simulink model "UTPR_MPC_LPV_22"  (R2023b)
settings: Solver=ode4  StartTime=0  StopTime=6  FixedStep=0.01  RelTol=1e-2  AbsTol=1e-3  EnableMultiTasking=on
values from neighbouring files (symbols this model uses):
  H = 0.05    [utpr_model_complex_para.m]    (also in utpr_mpc.m = (H + H')/2)
  L1 = 0.325    [utpr_model_complex_para.m]
  L2 = 0.2    [utpr_model_complex_para.m]
  L3 = 0.2    [utpr_model_complex_para.m]
  link1_CM = [245.436 * 1e-3 0 0]    [utpr_model_complex_para.m]
  link1_m = 1.915 * (rand_para(1,1) + 1)    [utpr_model_complex_para.m]
  link1_MI = [0 0 25720.752*1e-6* (rand_para(2,1) + 1)]    [utpr_model_complex_para.m]
  link1_PI = [0 0 0]    [utpr_model_complex_para.m]
  link2_CM = [165.468 * 1e-3 0 0]    [utpr_model_complex_para.m]
  link2_m = 1.469 * (rand_para(3,1) + 1)    [utpr_model_complex_para.m]
  link2_MI = [0 0 7667.511*1e-6* (rand_para(4,1) + 1)]    [utpr_model_complex_para.m]
  link2_PI = [0 0 0]    [utpr_model_complex_para.m]
  link3_CM = [127.337*1e-3 0 0]    [utpr_model_complex_para.m]
  link3_m = 1.141 * (rand_para(5,1) + 1)    [utpr_model_complex_para.m]
  link3_MI = [0 0 4949.014*1e-6* (rand_para(6,1) + 1)]    [utpr_model_complex_para.m]
  link3_PI = [0 0 0 ]    [utpr_model_complex_para.m]
  N = 50    [utpr_lqr.m]    (also in utpr_mpc.m = 100)
  W = 0.05    [utpr_model_complex_para.m]
undefined symbols (not defined in the file or in its folder): X, Y, Z
libraries: nesl_utility x24, sm_lib x17
settings Model: Creator=李东昊  LastModifiedBy=12720
settings SolverCC: AutoScaleAbsTol=off  AlgebraicLoopSolver=TrustRegion  MaxZcPerStep=1
settings DataIOCC: LimitDataPoints=on  MaxDataPoints=10000
settings OptimizationCC: ReuseModelBlockBuffer=off  LifeSpan=inf
settings DebuggingCC: UnconnectedInputMsg=warning  UnconnectedOutputMsg=warning  UnconnectedLineMsg=warning  AllowSymbolicDim=off  SFUnexpectedBacktrackingDiag=warning  SFNoUnconditionalDefaultTransitionDiag=warning  SFExecutionAtInitializationDiag=none  ArithmeticOperatorsInVariantConditions=warning
settings ModelReferenceCC: EnableRefExpFcnMdlSchedulingChecks=on
settings SFSimCC: SimUseLocalCustomCode=off  CustomCodeUndefinedFunction=UseInterfaceOnly
settings RTWCC: RTWUseLocalCustomCode=off  DLArmComputeVersion=19.05
settings CodeAppCC: StateflowObjectComments=on
settings GRTTargetCC: TargetLangStandard=C89/C90 (ANSI)
settings ConfigComp: CovMetricSettings=dw  CovSaveCumulativeToWorkspaceVar=on  CovSaveSingleToWorkspaceVar=on  CovExternalEMLEnable=off  CovSFcnEnable=off
settings SimscapeCC: SimscapeLogType=all  SimscapeLogSimulationStatistics=on  SimscapeLogDataHistory=10000
settings ExplorerConfigSet: InternalSimMechanicsExplorerSettings="<ExplorerConfiguration><canonicalview>aerospace</canonicalview><AnimationSetting><BasePlaybackSpeed>1.0</BasePlaybackSpeed><PlaybackSpeedFactor>1.0</PlaybackSpeedFactor></AnimationSetting><TilePanel><TileInfo><Tiles Columns=\"1\" Count=\"1\" Rows=\"1\"><Column Weight=\"1\"/><Row Weight=\"1\"/><Tile Height=\"1\" Width=\"1\" X=\"0\" Y=\"0\"/></Tiles></TileInfo><SceneInfo><SceneViewer><BGColor><R>0.60000002384185791</R><G>0.60000002384185791</G><B>0.60000002384185791</B></BGColor><Camera><DoPerspective>off</DoPerspective><Position><X>-0.471212034882517727</X><Y>0.213512906624389098</Y><Z>1.00000005247557366</Z></Position><Center><X>-0.471212034882517727</X><Y>0.213512906624389098</Y><Z>5.24755735531456935e-08</Z></Center><Up><X>0</X><Y>1</Y><Z>0</Z></Up><ViewLimDist>1</ViewLimDist><YLim>1.41406501065933288</YLim><XLim>1.62924881662923138</XLim></Camera></SceneViewer></SceneInfo></TilePanel><MechEditorPanel><Cameras/><GfxPanelCameraMap/><VideoCreator><PlaybackSpeedRatio>1.0</PlaybackSpeedRatio><FrameRate>30</FrameRate><VideoFormat>MPEG-4</VideoFormat><FrameSize>[800 600]</FrameSize></VideoCreator></MechEditorPanel></ExplorerConfiguration>"

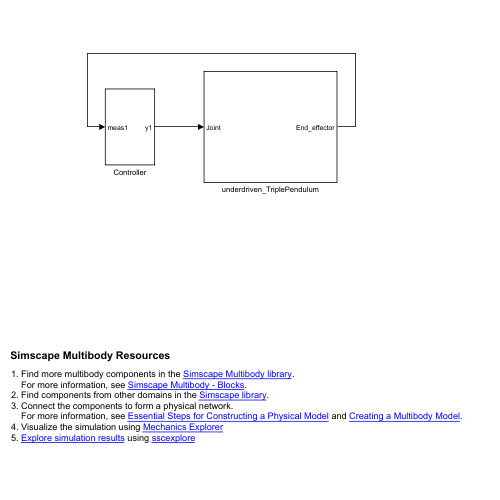
[thumbnail: Simulink's stored preview of the top-level diagram]
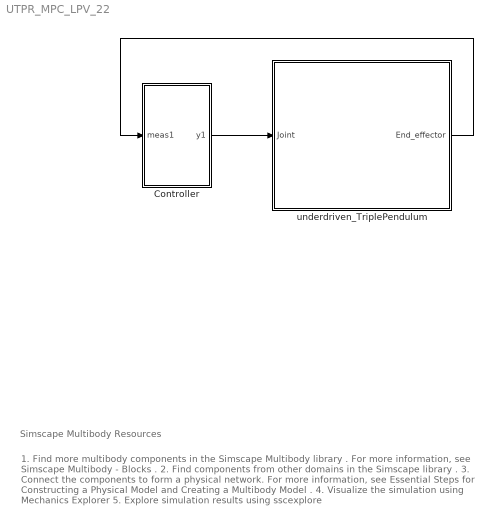
== system UTPR_MPC_LPV_22 ==
  note: 1. Find more multibody components in the Simscape Multibody library .
      | For more information, see Simscape Multibody - Blocks .
      | 2. Find components from other domains in the Simscape library .
      | 3. Connect the components to form a physical network.
      | For more information, see Essential Steps for Constructing a Physical Model and Creating a Multibody Model .
      | 4. Visualize the simulation using Mechanics Explorer
      | 5. Explore simulation results using sscexplore
  note: Simscape Multibody Resources
  Controller : Subsystem  Priority=1
  underdriven_TriplePendulum : Subsystem  Priority=2
  wires:
  underdriven_TriplePendulum/1(End_effector) -> Controller/1(meas1)
  Controller/1(y1) -> underdriven_TriplePendulum/1(Joint)

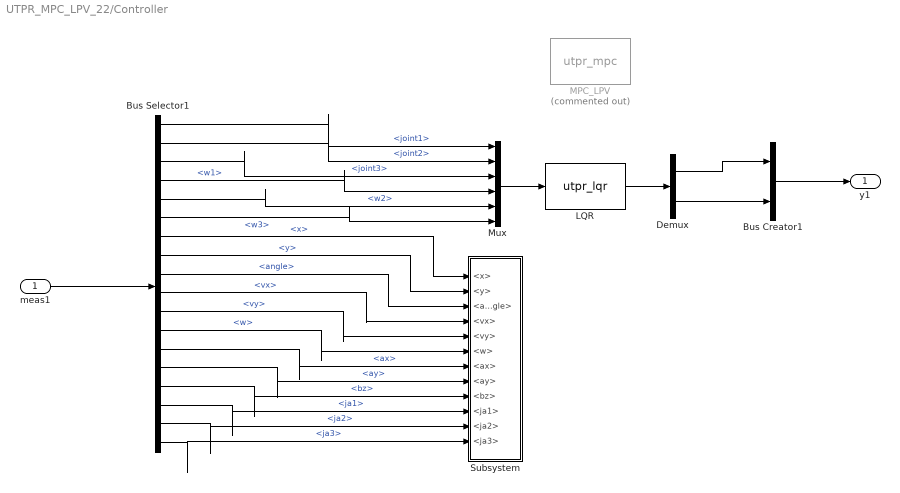
== system UTPR_MPC_LPV_22/Controller ==
  meas1 : Inport
  Bus Creator1 : BusCreator  Inputs=2
  Bus Selector1 : BusSelector  OutputSignals=joint1,joint2,joint3,w1,w2,w3,signal1.x,signal1.y,signal1.angle,signal1.vx,signal1.vy,signal1.w,signal1.ax,signal1.ay,signal1.bz,ja1,ja2,ja3
  Demux : Demux  Outputs=2
  LQR : MATLABFcn  MATLABFcn=utpr_lqr  OutputDimensions=2
  MPC_LPV : MATLABFcn  Commented=on  MATLABFcn=utpr_mpc  OutputDimensions=2
  Mux : Mux  Inputs=6
  Subsystem : Subsystem
  y1 : Outport
  wires:
  Bus Creator1/1 -> y1/1
  meas1/1 -> Bus Selector1/1
  Bus Selector1/1 -> Mux/1  "<joint1>"
  Bus Selector1/2 -> Mux/2  "<joint2>"
  Bus Selector1/3 -> Mux/3  "<joint3>"
  Bus Selector1/4 -> Mux/4  "<w1>"
  Bus Selector1/6 -> Mux/6  "<w3>"
  Demux/1 -> Bus Creator1/1
  Demux/2 -> Bus Creator1/2
  Bus Selector1/7 -> Subsystem/1(<x>)  "<x>"
  Bus Selector1/8 -> Subsystem/2(<y>)  "<y>"
  Bus Selector1/9 -> Subsystem/3(<angle>)  "<angle>"
  Bus Selector1/10 -> Subsystem/4(<vx>)  "<vx>"
  Bus Selector1/11 -> Subsystem/5(<vy>)  "<vy>"
  Bus Selector1/12 -> Subsystem/6(<w>)  "<w>"
  Bus Selector1/13 -> Subsystem/7(<ax>)  "<ax>"
  Bus Selector1/14 -> Subsystem/8(<ay>)  "<ay>"
  Bus Selector1/15 -> Subsystem/9(<bz>)  "<bz>"
  Bus Selector1/16 -> Subsystem/10(<ja1>)  "<ja1>"
  Bus Selector1/17 -> Subsystem/11(<ja2>)  "<ja2>"
  Bus Selector1/18 -> Subsystem/12(<ja3>)  "<ja3>"
  Bus Selector1/5 -> Mux/5  "<w2>"
  Mux/1 -> LQR/1
  LQR/1 -> Demux/1

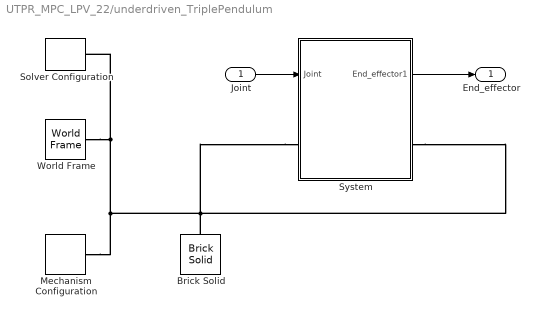
== system UTPR_MPC_LPV_22/underdriven_TriplePendulum ==
  Joint : Inport
  Brick Solid : sm_lib/Body Elements/Brick Solid  BrickDimensions=[0.1 0.1 0.1]  BrickDimensionsUnits=m  ExportEntireGeometry=off  InertiaType=CalculateFromGeometry  BasedOnType=Density  Density=1000  DensityUnits=kg/m^3  Mass=1  MassUnits=kg  CenterOfMass=[0 0 0]  CenterOfMassUnits=m  MomentsOfInertia=[1 1 1]  MomentsOfInertiaUnits=kg*m^2  ProductsOfInertia=[0 0 0]  ProductsOfInertiaUnits=kg*m^2  GraphicType=FromGeometry  MarkerShape=Sphere  MarkerSize=10  GraphicVisPropType=SimpleVisualProperties  GraphicDiffuseColor=[0.5 0.5 0.5]  GraphicOpacity=1.0  GraphicSpecularColor=[0.5 0.5 0.5 1.0]  GraphicAmbientColor=[0.15 0.15 0.15 1.0]  GraphicEmissiveColor=[0.0 0.0 0.0 1.0]  GraphicShininess=75  DoExposeReferenceFrame=on  SerializedFrames=<Frames/>
  Mechanism Configuration : sm_lib/Utilities/Mechanism Configuration  UniformGravity=Constant  GravityVector=[0 -9.81 0]  GravityVectorUnits=m/s^2  LinearizationDelta=0.001  JointModeTransitionNonlinearIterations=2
  Solver Configuration : nesl_utility/Solver Configuration  PhysicalDomain=network_engine_domain  SubClassName=solver  LeftPortType=input  RightPortType=generic  Tones=[]  Harmonics=[]  SimulateNoise=off  Profile=off  UseLocalSampling=off  EnableSwitchedLinearOptims=on  FrequencyDomain=off  UseCCode=off  RelTol=0.001  AbsTol=1e-06  MinStep=1e-09  ToWorkspace=off  RevertToSquareIcSolve=off  NumHomotopyIterations=100  PhasorMode=off  PhasorModeNumHarmonics=1  ConsistencySolver=NEWTON_FTOL  IndexReductionMethod=DerivativeReplacement  DoDC=off  ResidualTolerance=1e-09  ConsistencyTolSource=GLOBAL  ConsistencyAbsTol=0.001  ConsistencyRelTol=0.001  ConsistencyTolFactor=0.001  UseLocalSolver=off  LocalSolverChoice=NE_BACKWARD_EULER_ADVANCER  ResolveIndetEquations=on  FunctionEvalNumThread=1  LocalSolverSampleTime=0.001  DoFixedCost=off  MaxNonlinIter=3  MaxModeIter=2  ComputeImpulses=off  ImpulseIterations=2  LinearAlgebra=Sparse  LinearAlgebraNumThread=0  EquationFormulation=NE_TIME_EF  DelaysMemoryBudget=1024  AutomaticFiltering=on  FilteringTimeConstant=0.001  PartitionStorageMethod=AS_NEEDED  PartitionMemoryBudget=1024  PartitionMethod=FAST  MultibodyUseLocalSolver=off  MultibodyLocalSolverChoice=ODE1  MultibodyLocalSolverSampleTime=0.001
  System : Subsystem
  World Frame : sm_lib/Frames and Transforms/World Frame
  End_effector : Outport
  wires:
  Joint/1 -> System/1(Joint)
  System/1(End_effector1) -> End_effector/1
  connections:
  System/LConn1 -- World Frame/RConn1 -- Solver Configuration/RConn1 -- Mechanism Configuration/RConn1 -- Brick Solid/RConn1 -- System/RConn1

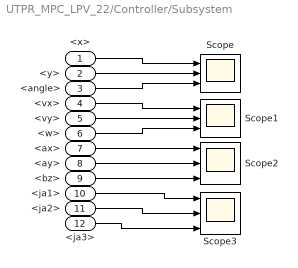
== system UTPR_MPC_LPV_22/Controller/Subsystem ==
  <x> : Inport
  <y> : Inport  Port=2
  <angle> : Inport  Port=3
  <vx> : Inport  Port=4
  <vy> : Inport  Port=5
  <w> : Inport  Port=6
  <ax> : Inport  Port=7
  <ay> : Inport  Port=8
  <bz> : Inport  Port=9
  <ja1> : Inport  Port=10
  <ja2> : Inport  Port=11
  <ja3> : Inport  Port=12
  Scope{,1..3} (4 alike) : Scope  NumInputPorts=3
  wires:
  <y>/1 -> Scope/2
  <ja1>/1 -> Scope3/1
  <bz>/1 -> Scope2/3
  <ax>/1 -> Scope2/1
  <vy>/1 -> Scope1/2
  <x>/1 -> Scope/1
  <angle>/1 -> Scope/3
  <ja2>/1 -> Scope3/2
  <ay>/1 -> Scope2/2
  <w>/1 -> Scope1/3
  <vx>/1 -> Scope1/1
  <ja3>/1 -> Scope3/3

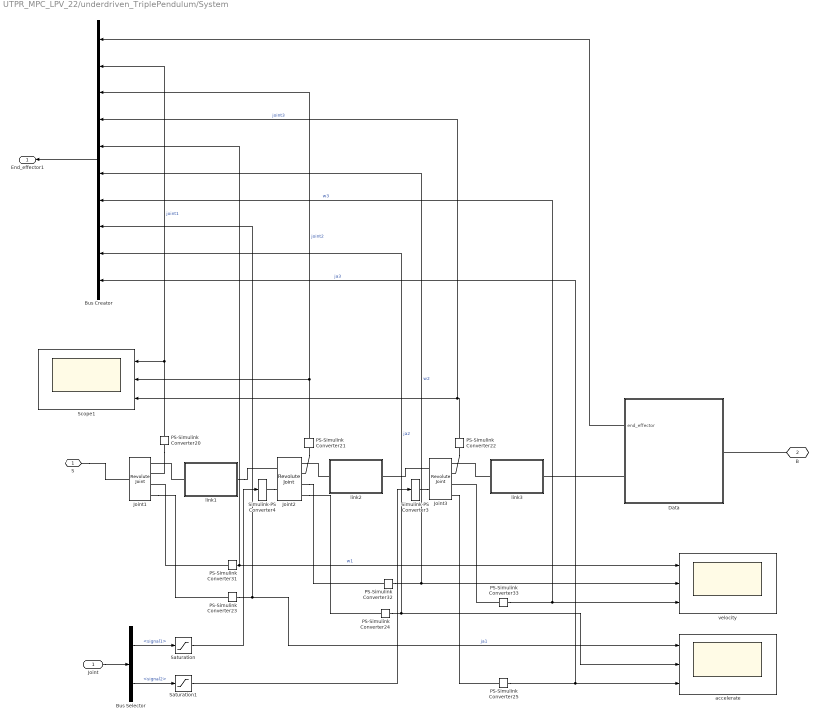
== system UTPR_MPC_LPV_22/underdriven_TriplePendulum/System ==
  Joint : Inport
  Bus Creator : BusCreator  Inputs=10
  Bus Selector : BusSelector  OutputSignals=signal1,signal2
  Data : Subsystem
  Joint1 : sm_lib/Joints/Revolute Joint  JointMode=Normal  CompositeWrenchDir=BaseOnFollower  CompositeWrenchFrame=BaseFrame  SenseConstraintForce=off  SenseConstraintTorque=off  SenseTotalForce=off  SenseTotalTorque=off  PositionTargetSpecify=on  PositionTargetPriority=High  PositionTargetValue=0.9  PositionTargetValueUnits=deg  VelocityTargetSpecify=off  VelocityTargetPriority=Low  VelocityTargetValue=0  VelocityTargetValueUnits=rad/s  EquilibriumPosition=0  EquilibriumPositionUnits=deg  SpringStiffness=0  SpringStiffnessUnits=N*m/deg  DampingCoefficient=0  DampingCoefficientUnits=N*m/(deg/s)  LowerLimitSpecify=off  LowerLimitBound=-90  LowerLimitBoundUnits=deg  LowerLimitStiffness=1e4  LowerLimitStiffnessUnits=N*m/deg  LowerLimitDamping=10  LowerLimitDampingUnits=N*m/(deg/s)  LowerLimitTransitionRegionWidth=0.1  LowerLimitTransitionRegionWidthUnits=deg  UpperLimitSpecify=off  UpperLimitBound=90  UpperLimitBoundUnits=deg  UpperLimitStiffness=1e4  UpperLimitStiffnessUnits=N*m/deg  UpperLimitDamping=10  UpperLimitDampingUnits=N*m/(deg/s)  UpperLimitTransitionRegionWidth=0.1  UpperLimitTransitionRegionWidthUnits=deg  TorqueActuationMode=NoTorque  MotionActuationMode=ComputedMotion  SensePosition=on  SenseVelocity=on  SenseAcceleration=on  SenseTorqueForce=off  SenseLowerLimitTorqueForce=off  SenseUpperLimitTorqueForce=off
  Joint2 : sm_lib/Joints/Revolute Joint  JointMode=Normal  CompositeWrenchDir=BaseOnFollower  CompositeWrenchFrame=BaseFrame  SenseConstraintForce=off  SenseConstraintTorque=off  SenseTotalForce=off  SenseTotalTorque=off  PositionTargetSpecify=on  PositionTargetPriority=High  PositionTargetValue=0.9  PositionTargetValueUnits=deg  VelocityTargetSpecify=off  VelocityTargetPriority=High  VelocityTargetValue=0  VelocityTargetValueUnits=rad/s  EquilibriumPosition=0  EquilibriumPositionUnits=deg  SpringStiffness=0  SpringStiffnessUnits=N*m/deg  DampingCoefficient=0  DampingCoefficientUnits=N*m/(deg/s)  LowerLimitSpecify=off  LowerLimitBound=-90  LowerLimitBoundUnits=rad  LowerLimitStiffness=0  LowerLimitStiffnessUnits=N*m/deg  LowerLimitDamping=0  LowerLimitDampingUnits=N*m/(deg/s)  LowerLimitTransitionRegionWidth=0.0  LowerLimitTransitionRegionWidthUnits=deg  UpperLimitSpecify=off  UpperLimitBound=90  UpperLimitBoundUnits=deg  UpperLimitStiffness=1e4  UpperLimitStiffnessUnits=N*m/deg  UpperLimitDamping=10  UpperLimitDampingUnits=N*m/(deg/s)  UpperLimitTransitionRegionWidth=0.1  UpperLimitTransitionRegionWidthUnits=deg  TorqueActuationMode=InputTorque  MotionActuationMode=ComputedMotion  SensePosition=on  SenseVelocity=on  SenseAcceleration=on  SenseTorqueForce=off  SenseLowerLimitTorqueForce=off  SenseUpperLimitTorqueForce=off
  Joint3 : sm_lib/Joints/Revolute Joint  JointMode=Normal  CompositeWrenchDir=BaseOnFollower  CompositeWrenchFrame=BaseFrame  SenseConstraintForce=off  SenseConstraintTorque=off  SenseTotalForce=off  SenseTotalTorque=off  PositionTargetSpecify=on  PositionTargetPriority=High  PositionTargetValue=0.9  PositionTargetValueUnits=deg  VelocityTargetSpecify=off  VelocityTargetPriority=High  VelocityTargetValue=0  VelocityTargetValueUnits=rad/s  EquilibriumPosition=0  EquilibriumPositionUnits=deg  SpringStiffness=0  SpringStiffnessUnits=N*m/deg  DampingCoefficient=0  DampingCoefficientUnits=N*m/(deg/s)  LowerLimitSpecify=off  LowerLimitBound=-90  LowerLimitBoundUnits=deg  LowerLimitStiffness=1e4  LowerLimitStiffnessUnits=N*m/deg  LowerLimitDamping=10  LowerLimitDampingUnits=N*m/(deg/s)  LowerLimitTransitionRegionWidth=0.1  LowerLimitTransitionRegionWidthUnits=deg  UpperLimitSpecify=off  UpperLimitBound=90  UpperLimitBoundUnits=deg  UpperLimitStiffness=1e4  UpperLimitStiffnessUnits=N*m/deg  UpperLimitDamping=10  UpperLimitDampingUnits=N*m/(deg/s)  UpperLimitTransitionRegionWidth=0.1  UpperLimitTransitionRegionWidthUnits=deg  TorqueActuationMode=InputTorque  MotionActuationMode=ComputedMotion  SensePosition=on  SenseVelocity=on  SenseAcceleration=on  SenseTorqueForce=off  SenseLowerLimitTorqueForce=off  SenseUpperLimitTorqueForce=off
  PS-Simulink Converter{20..25,31..33} (9 alike) : nesl_utility/PS-Simulink Converter  PhysicalDomain=network_engine_domain  SubClassName=ps_output  LeftPortType=input  RightPortType=output  PseudoPeriodic=off  Frequencies=[]  VectorFormat=inherit  Unit=inherit  AffineConversion=off
  Saturation : Saturate  UpperLimit=3  LowerLimit=-3
  Saturation1 : Saturate  UpperLimit=3  LowerLimit=-3
  Scope1 : Scope  NumInputPorts=3
  Simulink-PS Converter3 : nesl_utility/Simulink-PS Converter  PhysicalDomain=network_engine_domain  SubClassName=ps_input  LeftPortType=input  RightPortType=output  PseudoPeriodic=off  Frequencies=[]  NoiseDistribution=none  NoiseParameters=[]  Unit=1  AffineConversion=off  FilteringAndDerivatives=provide  SimscapeFilterOrder=2  InputFilterTimeConstant=0.001  UdotUserProvided=0
  Simulink-PS Converter4 : nesl_utility/Simulink-PS Converter  PhysicalDomain=network_engine_domain  SubClassName=ps_input  LeftPortType=input  RightPortType=output  PseudoPeriodic=off  Frequencies=[]  NoiseDistribution=none  NoiseParameters=[]  Unit=1  AffineConversion=off  FilteringAndDerivatives=provide  SimscapeFilterOrder=2  InputFilterTimeConstant=0.001  UdotUserProvided=0
  accelerate : Scope  NumInputPorts=3
  link1 : Subsystem  mask{L=L1, H=H, W=W, m=link1_m, link1_CM=link1_CM, link1_MI=link1_MI, link1_PI=link1_PI, rgb=[0.2 0.3 0.4]}
      mask prompts: link1_CM "Center of Mass"; link1_MI "Moments of Inertia"; link1_PI "Products of Inertia"; rgb "Color"
      mask DialogControl ParameterGroupVar Prompt: 参数
  link2 : Subsystem  mask{L=L2, W=W, H=W, llink2_m=link2_m, link2_CM=link2_CM, link2_MI=link2_MI, link2_PI=link2_PI, rgb=[1 1 0]}
      mask prompts: llink2_m "m(kg)"; link2_CM "Center of Mass"; link2_MI "Moments of Inertia"; link2_PI "Products of Inertia"
      mask DialogControl ParameterGroupVar Prompt: 参数
  link3 : Subsystem  mask{L=L3, W=W, H=H, link3_m=link3_m, link3_CM=link3_CM, link3_MI=link3_MI, link3_PI=link3_PI, rgb=[1 0.40 0.00]}
      mask prompts: link3_m "m"; link3_CM "Center of Mass"; link3_MI "Moments of Inertia"; link3_PI "Product of Inertia"
      mask DialogControl ParameterGroupVar Prompt: 参数
  velocity : Scope  NumInputPorts=3
  S : PMIOPort  Side=Left
  B : PMIOPort  Port=2  Side=Right
  End_effector1 : Outport
  wires:
  PS-Simulink Converter24/1 -> accelerate/2, Bus Creator/9  "ja2"
  PS-Simulink Converter32/1 -> Bus Creator/6, velocity/2  "w2"
  PS-Simulink Converter25/1 -> Bus Creator/10, accelerate/3  "ja3"
  PS-Simulink Converter22/1 -> Bus Creator/4, Scope1/3  "joint3"
  PS-Simulink Converter20/1 -> Bus Creator/2, Scope1/1  "joint1"
  Bus Selector/2 -> Saturation1/1  "<signal2>"
  PS-Simulink Converter21/1 -> Bus Creator/3, Scope1/2  "joint2"
  Bus Selector/1 -> Saturation/1  "<signal1>"
  PS-Simulink Converter33/1 -> Bus Creator/7, velocity/3  "w3"
  PS-Simulink Converter31/1 -> Bus Creator/5, velocity/1  "w1"
  Joint/1 -> Bus Selector/1
  Data/1(end_effector) -> Bus Creator/1
  Bus Creator/1 -> End_effector1/1
  PS-Simulink Converter23/1 -> accelerate/1, Bus Creator/8  "ja1"
  Saturation/1 -> Simulink-PS Converter4/1
  Saturation1/1 -> Simulink-PS Converter3/1
  connections:
  PS-Simulink Converter21/LConn1 -- Joint2/RConn2
  Joint2/RConn4 -- PS-Simulink Converter24/LConn1
  Joint3/RConn4 -- PS-Simulink Converter25/LConn1
  PS-Simulink Converter20/LConn1 -- Joint1/RConn2
  link1/LConn1 -- Joint1/RConn1
  PS-Simulink Converter22/LConn1 -- Joint3/RConn2
  link1/RConn1 -- Joint2/LConn1
  Simulink-PS Converter3/RConn1 -- Joint3/LConn2
  Joint1/RConn4 -- PS-Simulink Converter23/LConn1
  PS-Simulink Converter33/LConn1 -- Joint3/RConn3
  PS-Simulink Converter31/LConn1 -- Joint1/RConn3
  link3/LConn1 -- Joint3/RConn1
  S/RConn1 -- Joint1/LConn1
  link2/LConn1 -- Joint2/RConn1
  Joint3/LConn1 -- link2/RConn1
  Simulink-PS Converter4/RConn1 -- Joint2/LConn2
  Joint2/RConn3 -- PS-Simulink Converter32/LConn1
  B/RConn1 -- Data/LConn1
  Data/RConn1 -- link3/RConn1

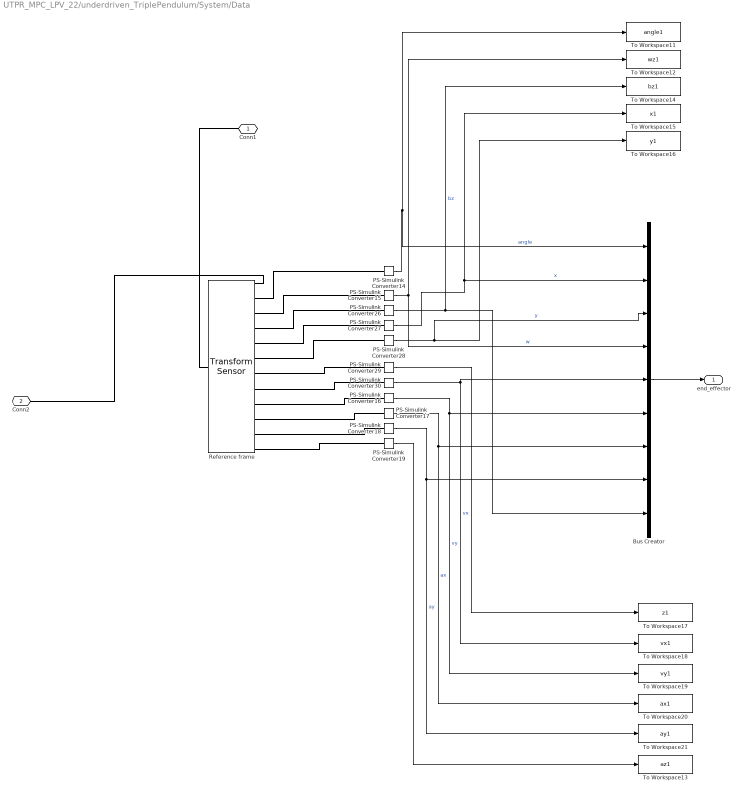
== system UTPR_MPC_LPV_22/underdriven_TriplePendulum/System/Data ==
  Bus Creator : BusCreator  Inputs=9
  PS-Simulink Converter{14..19,26..30} (11 alike) : nesl_utility/PS-Simulink Converter  PhysicalDomain=network_engine_domain  SubClassName=ps_output  LeftPortType=input  RightPortType=output  PseudoPeriodic=off  Frequencies=[]  VectorFormat=inherit  Unit=inherit  AffineConversion=off
  Reference frame : sm_lib/Frames and Transforms/Transform Sensor  MeasurementFrame=Base  RotationSequence=XYX  SenseAngle=on  SenseAxis=off  SenseQ=off  SenseR=off  SenseRotationSequence=off  SenseOmegaX=off  SenseOmegaY=off  SenseOmegaZ=on  SenseOmega=off  SenseQDot=off  SenseRDot=off  SenseRotationSequenceDot=off  SenseAlphaX=off  SenseAlphaY=off  SenseAlphaZ=on  SenseAlpha=off  SenseQDDot=off  SenseRDDot=off  SenseX=on  SenseY=on  SenseZ=on  SenseXYZ=off  SenseRad=off  SenseAzim=off  SenseDist=off  SenseInc=off  SenseXDot=on  SenseYDot=on  SenseZDot=off  SenseXYZDot=off  SenseRadDot=off  SenseAzimDot=off  SenseDistDot=off  SenseIncDot=off  SenseXDDot=on  SenseYDDot=on  SenseZDDot=on  SenseXYZDDot=off  SenseRadDDot=off  SenseAzimDDot=off  SenseDistDDot=off  SenseIncDDot=off
  To Workspace11 : ToWorkspace  VariableName=angle1  SaveFormat=Structure With Time  SampleTime=-1
  To Workspace12 : ToWorkspace  VariableName=wz1  SaveFormat=Structure With Time  SampleTime=-1
  To Workspace13 : ToWorkspace  VariableName=az1  SaveFormat=Structure With Time  SampleTime=-1
  To Workspace14 : ToWorkspace  VariableName=bz1  SaveFormat=Structure With Time  SampleTime=-1
  To Workspace15 : ToWorkspace  VariableName=x1  SaveFormat=Structure With Time  SampleTime=-1
  To Workspace16 : ToWorkspace  VariableName=y1  SaveFormat=Structure With Time  SampleTime=-1
  To Workspace17 : ToWorkspace  VariableName=z1  SaveFormat=Structure With Time  SampleTime=-1
  To Workspace18 : ToWorkspace  VariableName=vx1  SaveFormat=Structure With Time  SampleTime=-1
  To Workspace19 : ToWorkspace  VariableName=vy1  SaveFormat=Structure With Time  SampleTime=-1
  To Workspace20 : ToWorkspace  VariableName=ax1  SaveFormat=Structure With Time  SampleTime=-1
  To Workspace21 : ToWorkspace  VariableName=ay1  SaveFormat=Structure With Time  SampleTime=-1
  Conn1 : PMIOPort  Side=Left
  Conn2 : PMIOPort  Port=2  Side=Right
  end_effector : Outport
  wires:
  PS-Simulink Converter26/1 -> Bus Creator/9, To Workspace14/1  "bz"
  PS-Simulink Converter17/1 -> Bus Creator/7, To Workspace20/1  "ax"
  PS-Simulink Converter18/1 -> Bus Creator/8, To Workspace21/1  "ay"
  PS-Simulink Converter15/1 -> To Workspace12/1, Bus Creator/4  "w"
  PS-Simulink Converter27/1 -> Bus Creator/2, To Workspace15/1  "x"
  PS-Simulink Converter29/1 -> To Workspace17/1
  PS-Simulink Converter19/1 -> To Workspace13/1
  PS-Simulink Converter14/1 -> Bus Creator/1, To Workspace11/1  "angle"
  PS-Simulink Converter16/1 -> To Workspace19/1, Bus Creator/6  "vy"
  PS-Simulink Converter28/1 -> To Workspace16/1, Bus Creator/3  "y"
  PS-Simulink Converter30/1 -> To Workspace18/1, Bus Creator/5  "vx"
  Bus Creator/1 -> end_effector/1
  connections:
  Reference frame/RConn3 -- PS-Simulink Converter15/LConn1
  Reference frame/RConn7 -- PS-Simulink Converter29/LConn1
  Reference frame/RConn6 -- PS-Simulink Converter28/LConn1
  Reference frame/RConn8 -- PS-Simulink Converter30/LConn1
  Reference frame/RConn9 -- PS-Simulink Converter16/LConn1
  Reference frame/RConn11 -- PS-Simulink Converter18/LConn1
  Reference frame/RConn4 -- PS-Simulink Converter26/LConn1
  PS-Simulink Converter14/LConn1 -- Reference frame/RConn2
  Reference frame/RConn10 -- PS-Simulink Converter17/LConn1
  Reference frame/RConn5 -- PS-Simulink Converter27/LConn1
  Reference frame/RConn1 -- Conn2/RConn1
  Conn1/RConn1 -- Reference frame/LConn1
  Reference frame/RConn12 -- PS-Simulink Converter19/LConn1

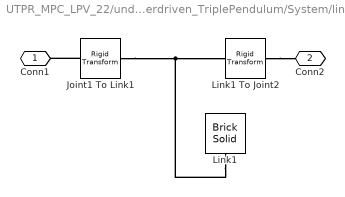
== system UTPR_MPC_LPV_22/underdriven_TriplePendulum/System/link1 ==
  Joint1 To Link1 : sm_lib/Frames and Transforms/Rigid Transform  RotationMethod=StandardAxis  FollAlignAxisA=+X  BaseAlignAxisA=+Y  FollAlignAxisB=+Y  BaseAlignAxisB=+Z  RotationStandardAxis=+Z  RotationAngle=90  RotationAngleUnits=deg  RotationArbitraryAxis=[0 0 1]  RotationSequenceAxes=FollowerAxes  RotationSequence=XYX  RotationSequenceAngles=[0 0 0]  RotationSequenceAnglesUnits=deg  RotationMatrix=[1 0 0; 0 1 0; 0 0 1]  Quaternion=[1 0 0 0]  TranslationMethod=StandardAxis  TranslationCartesianOffset=[0 0 0]  TranslationCartesianOffsetUnits=m  TranslationStandardAxis=+Y  TranslationStandardOffset=0  TranslationStandardOffsetUnits=m  TranslationROffset=0  TranslationROffsetUnits=m  TranslationThetaOffset=0  TranslationThetaOffsetUnits=deg  TranslationZOffset=0  TranslationZOffsetUnits=m
  Link1 : sm_lib/Body Elements/Brick Solid  BrickDimensions=[L H W]  BrickDimensionsUnits=m  ExportEntireGeometry=off  InertiaType=Custom  BasedOnType=Density  Density=rho  DensityUnits=kg/m^3  Mass=link1_m  MassUnits=kg  CenterOfMass=link1_CM  CenterOfMassUnits=m  MomentsOfInertia=link1_MI  MomentsOfInertiaUnits=kg*m^2  ProductsOfInertia=link1_PI  ProductsOfInertiaUnits=kg*m^2  GraphicType=FromGeometry  MarkerShape=Sphere  MarkerSize=10  GraphicVisPropType=SimpleVisualProperties  GraphicDiffuseColor=rgb  GraphicOpacity=1.0  GraphicSpecularColor=[0.5 0.5 0.5 1.0]  GraphicAmbientColor=[0.15 0.15 0.15 1.0]  GraphicEmissiveColor=[0.0 0.0 0.0 1.0]  GraphicShininess=75  DoExposeReferenceFrame=off  SerializedFrames=<Frames><Frame><Id>Frame1</Id><Value><Name>F1</Name><Origin><Source>GeometricFeature</Source><FeatureName>-x surface</FeatureName></Origin><PrimaryAxis><DefinedDirection>+Y</DefinedDirection><Source>ReferenceFrame</Source><SourceDirection>+Y</SourceDirection><FeatureName></FeatureName></PrimaryAxis><SecondaryAxis><DefinedDirection>+X</DefinedDirection><Source>ReferenceFrame</Source><SourceDirection>+X</SourceDirection><FeatureName></FeatureName></SecondaryAxis></Value></Frame></Frames>
  Link1 To Joint2 : sm_lib/Frames and Transforms/Rigid Transform  RotationMethod=None  FollAlignAxisA=+X  BaseAlignAxisA=+Y  FollAlignAxisB=+Y  BaseAlignAxisB=+Z  RotationStandardAxis=+Z  RotationAngle=0.0  RotationAngleUnits=deg  RotationArbitraryAxis=[0 0 1]  RotationSequenceAxes=FollowerAxes  RotationSequence=XYX  RotationSequenceAngles=[0 0 0]  RotationSequenceAnglesUnits=deg  RotationMatrix=[1 0 0; 0 1 0; 0 0 1]  Quaternion=[1 0 0 0]  TranslationMethod=StandardAxis  TranslationCartesianOffset=[0 0 0]  TranslationCartesianOffsetUnits=m  TranslationStandardAxis=+X  TranslationStandardOffset=L1  TranslationStandardOffsetUnits=m  TranslationROffset=0  TranslationROffsetUnits=m  TranslationThetaOffset=0  TranslationThetaOffsetUnits=deg  TranslationZOffset=0  TranslationZOffsetUnits=m
  Conn1 : PMIOPort  Side=Left
  Conn2 : PMIOPort  Port=2  Side=Right
  connections:
  Joint1 To Link1/RConn1 -- Link1/LConn1 -- Link1 To Joint2/LConn1
  Joint1 To Link1/LConn1 -- Conn1/RConn1
  Link1 To Joint2/RConn1 -- Conn2/RConn1

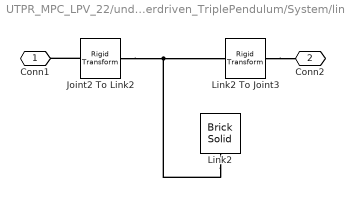
== system UTPR_MPC_LPV_22/underdriven_TriplePendulum/System/link2 ==
  Joint2 To Link2 : sm_lib/Frames and Transforms/Rigid Transform  RotationMethod=None  FollAlignAxisA=+X  BaseAlignAxisA=+Y  FollAlignAxisB=+Y  BaseAlignAxisB=+Z  RotationStandardAxis=+Z  RotationAngle=0.0  RotationAngleUnits=deg  RotationArbitraryAxis=[0 0 1]  RotationSequenceAxes=FollowerAxes  RotationSequence=XYX  RotationSequenceAngles=[0 0 0]  RotationSequenceAnglesUnits=deg  RotationMatrix=[1 0 0; 0 1 0; 0 0 1]  Quaternion=[1 0 0 0]  TranslationMethod=StandardAxis  TranslationCartesianOffset=[0 0 0]  TranslationCartesianOffsetUnits=m  TranslationStandardAxis=+X  TranslationStandardOffset=0  TranslationStandardOffsetUnits=m  TranslationROffset=0  TranslationROffsetUnits=m  TranslationThetaOffset=0  TranslationThetaOffsetUnits=deg  TranslationZOffset=0  TranslationZOffsetUnits=m
  Link2 : sm_lib/Body Elements/Brick Solid  BrickDimensions=[L H W]  BrickDimensionsUnits=m  ExportEntireGeometry=off  InertiaType=Custom  BasedOnType=Density  Density=rho  DensityUnits=kg/m^3  Mass=link2_m  MassUnits=kg  CenterOfMass=link2_CM  CenterOfMassUnits=m  MomentsOfInertia=link2_MI  MomentsOfInertiaUnits=kg*m^2  ProductsOfInertia=link2_PI  ProductsOfInertiaUnits=kg*m^2  GraphicType=FromGeometry  MarkerShape=Sphere  MarkerSize=10  GraphicVisPropType=SimpleVisualProperties  GraphicDiffuseColor=rgb  GraphicOpacity=1.0  GraphicSpecularColor=[0.5 0.5 0.5 1.0]  GraphicAmbientColor=[0.15 0.15 0.15 1.0]  GraphicEmissiveColor=[0.0 0.0 0.0 1.0]  GraphicShininess=75  DoExposeReferenceFrame=off  SerializedFrames=<Frames><Frame><Id>Frame1</Id><Value><Name>F1</Name><Origin><Source>GeometricFeature</Source><FeatureName>-x surface</FeatureName></Origin><PrimaryAxis><DefinedDirection>+Z</DefinedDirection><Source>ReferenceFrame</Source><SourceDirection>+Z</SourceDirection><FeatureName></FeatureName></PrimaryAxis><SecondaryAxis><DefinedDirection>+X</DefinedDirection><Source>ReferenceFrame</Source><SourceDirection>+X</SourceDirection><FeatureName></FeatureName></SecondaryAxis></Value></Frame></Frames>
  Link2 To Joint3 : sm_lib/Frames and Transforms/Rigid Transform  RotationMethod=None  FollAlignAxisA=+X  BaseAlignAxisA=+Y  FollAlignAxisB=+Y  BaseAlignAxisB=+Z  RotationStandardAxis=+Z  RotationAngle=0.0  RotationAngleUnits=deg  RotationArbitraryAxis=[0 0 1]  RotationSequenceAxes=FollowerAxes  RotationSequence=XYX  RotationSequenceAngles=[0 0 0]  RotationSequenceAnglesUnits=deg  RotationMatrix=[1 0 0; 0 1 0; 0 0 1]  Quaternion=[1 0 0 0]  TranslationMethod=StandardAxis  TranslationCartesianOffset=[0 0 0]  TranslationCartesianOffsetUnits=m  TranslationStandardAxis=+X  TranslationStandardOffset=L2  TranslationStandardOffsetUnits=m  TranslationROffset=0  TranslationROffsetUnits=m  TranslationThetaOffset=0  TranslationThetaOffsetUnits=deg  TranslationZOffset=0  TranslationZOffsetUnits=m
  Conn1 : PMIOPort  Side=Left
  Conn2 : PMIOPort  Port=2  Side=Right
  connections:
  Joint2 To Link2/RConn1 -- Link2/LConn1 -- Link2 To Joint3/LConn1
  Joint2 To Link2/LConn1 -- Conn1/RConn1
  Link2 To Joint3/RConn1 -- Conn2/RConn1

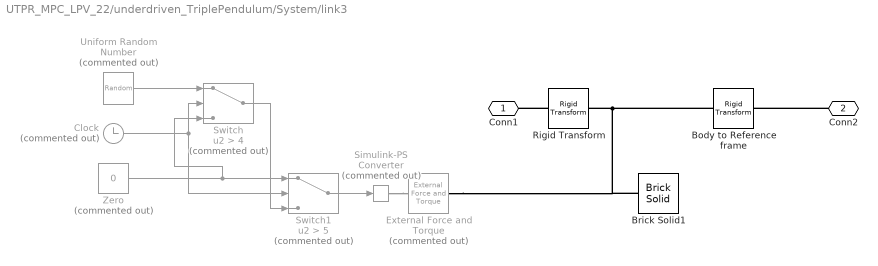
== system UTPR_MPC_LPV_22/underdriven_TriplePendulum/System/link3 ==
  Body to Reference frame : sm_lib/Frames and Transforms/Rigid Transform  RotationMethod=None  FollAlignAxisA=+X  BaseAlignAxisA=+Y  FollAlignAxisB=+Y  BaseAlignAxisB=+Z  RotationStandardAxis=-Z  RotationAngle=90  RotationAngleUnits=deg  RotationArbitraryAxis=[0 0 1]  RotationSequenceAxes=FollowerAxes  RotationSequence=XYX  RotationSequenceAngles=[0 0 0]  RotationSequenceAnglesUnits=deg  RotationMatrix=[1 0 0; 0 1 0; 0 0 1]  Quaternion=[1 0 0 0]  TranslationMethod=StandardAxis  TranslationCartesianOffset=[0 0 0]  TranslationCartesianOffsetUnits=m  TranslationStandardAxis=+X  TranslationStandardOffset=L3  TranslationStandardOffsetUnits=m  TranslationROffset=0  TranslationROffsetUnits=m  TranslationThetaOffset=0  TranslationThetaOffsetUnits=deg  TranslationZOffset=0  TranslationZOffsetUnits=m
  Brick Solid1 : sm_lib/Body Elements/Brick Solid  BrickDimensions=[L H W]  BrickDimensionsUnits=m  ExportEntireGeometry=off  InertiaType=Custom  BasedOnType=Density  Density=rho  DensityUnits=kg/m^3  Mass=link3_m  MassUnits=kg  CenterOfMass=link3_CM  CenterOfMassUnits=m  MomentsOfInertia=link3_MI  MomentsOfInertiaUnits=kg*m^2  ProductsOfInertia=link3_PI  ProductsOfInertiaUnits=kg*m^2  GraphicType=FromGeometry  MarkerShape=Sphere  MarkerSize=10  GraphicVisPropType=SimpleVisualProperties  GraphicDiffuseColor=rgb  GraphicOpacity=1.0  GraphicSpecularColor=[0.5 0.5 0.5 1.0]  GraphicAmbientColor=[0.15 0.15 0.15 1.0]  GraphicEmissiveColor=[0.0 0.0 0.0 1.0]  GraphicShininess=75  DoExposeReferenceFrame=off  SerializedFrames=<Frames><Frame><Id>Frame1</Id><Value><Name>F1</Name><Origin><Source>GeometricFeature</Source><FeatureName>-x surface</FeatureName></Origin><PrimaryAxis><DefinedDirection>+Z</DefinedDirection><Source>ReferenceFrame</Source><SourceDirection>+Z</SourceDirection><FeatureName></FeatureName></PrimaryAxis><SecondaryAxis><DefinedDirection>+X</DefinedDirection><Source>ReferenceFrame</Source><SourceDirection>+X</SourceDirection><FeatureName></FeatureName></SecondaryAxis></Value></Frame></Frames>
  Clock : Clock  Commented=on
  External Force and Torque : sm_lib/Forces and Torques/External Force and Torque  Commented=on  EnableForceX=on  EnableForceY=off  EnableForceZ=off  EnableForce=off  ForceResolutionFrame=World  EnableTorqueX=off  EnableTorqueY=off  EnableTorqueZ=off  EnableTorque=off  TorqueResolutionFrame=AttachedFrame
  Rigid Transform : sm_lib/Frames and Transforms/Rigid Transform  RotationMethod=None  FollAlignAxisA=+X  BaseAlignAxisA=+Y  FollAlignAxisB=+Y  BaseAlignAxisB=+Z  RotationStandardAxis=+Z  RotationAngle=0.0  RotationAngleUnits=deg  RotationArbitraryAxis=[0 0 1]  RotationSequenceAxes=FollowerAxes  RotationSequence=XYX  RotationSequenceAngles=[0 0 0]  RotationSequenceAnglesUnits=deg  RotationMatrix=[1 0 0; 0 1 0; 0 0 1]  Quaternion=[1 0 0 0]  TranslationMethod=StandardAxis  TranslationCartesianOffset=[0 0 0]  TranslationCartesianOffsetUnits=m  TranslationStandardAxis=+X  TranslationStandardOffset=0  TranslationStandardOffsetUnits=m  TranslationROffset=0  TranslationROffsetUnits=m  TranslationThetaOffset=0  TranslationThetaOffsetUnits=deg  TranslationZOffset=0  TranslationZOffsetUnits=m
  Simulink-PS Converter : nesl_utility/Simulink-PS Converter  Commented=on  PhysicalDomain=network_engine_domain  SubClassName=ps_input  LeftPortType=input  RightPortType=output  PseudoPeriodic=off  Frequencies=[]  NoiseDistribution=none  NoiseParameters=[]  Unit=1  AffineConversion=off  FilteringAndDerivatives=provide  SimscapeFilterOrder=1  InputFilterTimeConstant=0.001  UdotUserProvided=0
  Switch : Switch  Commented=on  Criteria=u2 > Threshold  Threshold=4  SaturateOnIntegerOverflow=off  InputSameDT=off
  Switch1 : Switch  Commented=on  Criteria=u2 > Threshold  Threshold=5  SaturateOnIntegerOverflow=off  InputSameDT=off
  Uniform Random Number : UniformRandomNumber  Commented=on  Minimum=-3.0  Maximum=3.0  SampleTime=0.001
  Zero : Constant  Commented=on  Value=0  OutDataTypeStr=Inherit: Inherit via back propagation
  Conn1 : PMIOPort  Side=Left
  Conn2 : PMIOPort  Port=2  Side=Right
  wires:
  Switch1/1 -> Simulink-PS Converter/1
  Clock/1 -> Switch1/2, Switch/2
  Zero/1 -> Switch1/1, Switch/3
  Uniform Random Number/1 -> Switch/1
  Switch/1 -> Switch1/3
  connections:
  Body to Reference frame/LConn1 -- External Force and Torque/RConn1 -- Brick Solid1/LConn1 -- Rigid Transform/RConn1
  Rigid Transform/LConn1 -- Conn1/RConn1
  Conn2/RConn1 -- Body to Reference frame/RConn1
  Simulink-PS Converter/RConn1 -- External Force and Torque/LConn1
